simulink model "MC33pwm"  (R2019a)
settings: Solver=ode23tb  StartTime=0.0  StopTime=0.2  RelTol=1e-3
libraries: powerlib x35
(part 2 of 2)

== system MC33pwm/Subsystem1/status/time xl/time xl pos/xl b_u ==
  In ABC : Inport
  In x : Inport  Port=2
  Logical Operator : Logic  Operator=NOT  AllPortsSameDT=off  OutDataTypeStr=boolean
  MinMax : MinMax
  Sign : Signum
  Sum : Sum  Inputs=|+-
  out xl_s12 : Outport
  wires:
  Sign/1 -> Logical Operator/1
  MinMax/1 -> Sum/1
  Logical Operator/1 -> out xl_s12/1
  In ABC/1 -> MinMax/1
  In x/1 -> Sum/2
  Sum/1 -> Sign/1

== system MC33pwm/Subsystem1/status/time xl/time xl pos/xl c_u ==
  In ABC : Inport
  In x : Inport  Port=2
  Logical Operator : Logic  Operator=NOT  AllPortsSameDT=off  OutDataTypeStr=boolean
  MinMax : MinMax
  Sign : Signum
  Sum : Sum  Inputs=|+-
  out xl_s13 : Outport
  wires:
  Sign/1 -> Logical Operator/1
  MinMax/1 -> Sum/1
  Logical Operator/1 -> out xl_s13/1
  In ABC/1 -> MinMax/1
  In x/1 -> Sum/2
  Sum/1 -> Sign/1

== system MC33pwm/Subsystem1/status/time zb/time zb neg/zb a_u ==
  In ABC : Inport
  In x : Inport  Port=2
  Logical Operator : Logic  Operator=NOT  AllPortsSameDT=off  OutDataTypeStr=boolean
  MinMax : MinMax  Function=max
  Sign : Signum
  Sum : Sum  Inputs=|+-
  out zb_s11 : Outport
  wires:
  MinMax/1 -> Sum/1
  In ABC/1 -> MinMax/1
  In x/1 -> Sum/2
  Sum/1 -> Sign/1
  Sign/1 -> Logical Operator/1
  Logical Operator/1 -> out zb_s11/1

== system MC33pwm/Subsystem1/status/time zb/time zb neg/zb b_u ==
  In ABC : Inport
  In x : Inport  Port=2
  Logical Operator : Logic  Operator=NOT  AllPortsSameDT=off  OutDataTypeStr=boolean
  MinMax : MinMax  Function=max
  Sign : Signum
  Sum : Sum  Inputs=|+-
  out zb_s12 : Outport
  wires:
  MinMax/1 -> Sum/1
  In ABC/1 -> MinMax/1
  In x/1 -> Sum/2
  Sum/1 -> Sign/1
  Logical Operator/1 -> out zb_s12/1
  Sign/1 -> Logical Operator/1

== system MC33pwm/Subsystem1/status/time zb/time zb neg/zb c_u ==
  In ABC : Inport
  In x : Inport  Port=2
  Logical Operator : Logic  Operator=NOT  AllPortsSameDT=off  OutDataTypeStr=boolean
  MinMax : MinMax  Function=max
  Sign : Signum
  Sum : Sum  Inputs=|+-
  out zb_s13 : Outport
  wires:
  MinMax/1 -> Sum/1
  In ABC/1 -> MinMax/1
  In x/1 -> Sum/2
  Sum/1 -> Sign/1
  Logical Operator/1 -> out zb_s13/1
  Sign/1 -> Logical Operator/1

== system MC33pwm/Subsystem1/status/time zb/time zb pos/zb a_u ==
  In ABC : Inport
  In x : Inport  Port=2
  Logical Operator : Logic  Operator=NOT  AllPortsSameDT=off  OutDataTypeStr=boolean
  MinMax : MinMax  Function=max
  Scope : Scope
  Sign : Signum
  Sum : Sum  Inputs=|+-
  out zb_s11 : Outport
  wires:
  Sign/1 -> Logical Operator/1
  MinMax/1 -> Sum/1
  Logical Operator/1 -> out zb_s11/1
  In ABC/1 -> MinMax/1
  In x/1 -> Sum/2
  Sum/1 -> Scope/1, Sign/1

== system MC33pwm/Subsystem1/status/time zb/time zb pos/zb b_u ==
  In ABC : Inport
  In x : Inport  Port=2
  Logical Operator : Logic  Operator=NOT  AllPortsSameDT=off  OutDataTypeStr=boolean
  MinMax : MinMax  Function=max
  Sign : Signum
  Sum : Sum  Inputs=|+-
  out zb_s12 : Outport
  wires:
  Sign/1 -> Logical Operator/1
  MinMax/1 -> Sum/1
  Logical Operator/1 -> out zb_s12/1
  In ABC/1 -> MinMax/1
  In x/1 -> Sum/2
  Sum/1 -> Sign/1

== system MC33pwm/Subsystem1/status/time zb/time zb pos/zb c_u ==
  In ABC : Inport
  In x : Inport  Port=2
  Logical Operator : Logic  Operator=NOT  AllPortsSameDT=off  OutDataTypeStr=boolean
  MinMax : MinMax  Function=max
  Sign : Signum
  Sum : Sum  Inputs=|+-
  out zb_s13 : Outport
  wires:
  Sign/1 -> Logical Operator/1
  MinMax/1 -> Sum/1
  Logical Operator/1 -> out zb_s13/1
  In ABC/1 -> MinMax/1
  In x/1 -> Sum/2
  Sum/1 -> Sign/1

== system MC33pwm/Subsystem2/status/time xl/time xl neg/xl a_u ==
  In ABC : Inport
  In x : Inport  Port=2
  Logical Operator : Logic  Operator=NOT  AllPortsSameDT=off  OutDataTypeStr=boolean
  MinMax : MinMax
  Sign : Signum
  Sum : Sum  Inputs=|+-
  out xl_s11 : Outport
  wires:
  MinMax/1 -> Sum/1
  In ABC/1 -> MinMax/1
  In x/1 -> Sum/2
  Sum/1 -> Sign/1
  Sign/1 -> Logical Operator/1
  Logical Operator/1 -> out xl_s11/1

== system MC33pwm/Subsystem2/status/time xl/time xl neg/xl b_u ==
  In ABC : Inport
  In x : Inport  Port=2
  Logical Operator : Logic  Operator=NOT  AllPortsSameDT=off  OutDataTypeStr=boolean
  MinMax : MinMax
  Sign : Signum
  Sum : Sum  Inputs=|+-
  out xl_s12 : Outport
  wires:
  MinMax/1 -> Sum/1
  In ABC/1 -> MinMax/1
  In x/1 -> Sum/2
  Sum/1 -> Sign/1
  Logical Operator/1 -> out xl_s12/1
  Sign/1 -> Logical Operator/1

== system MC33pwm/Subsystem2/status/time xl/time xl neg/xl c_u ==
  In ABC : Inport
  In x : Inport  Port=2
  Logical Operator : Logic  Operator=NOT  AllPortsSameDT=off  OutDataTypeStr=boolean
  MinMax : MinMax
  Sign : Signum
  Sum : Sum  Inputs=|+-
  out xl_s13 : Outport
  wires:
  MinMax/1 -> Sum/1
  In ABC/1 -> MinMax/1
  In x/1 -> Sum/2
  Sum/1 -> Sign/1
  Logical Operator/1 -> out xl_s13/1
  Sign/1 -> Logical Operator/1

== system MC33pwm/Subsystem2/status/time xl/time xl pos/xl a_u ==
  In ABC : Inport
  In x : Inport  Port=2
  Logical Operator : Logic  Operator=NOT  AllPortsSameDT=off  OutDataTypeStr=boolean
  MinMax : MinMax
  Scope : Scope
  Sign : Signum
  Sum : Sum  Inputs=|+-
  out xl_s11 : Outport
  wires:
  Sign/1 -> Logical Operator/1
  MinMax/1 -> Sum/1
  Logical Operator/1 -> out xl_s11/1
  In ABC/1 -> MinMax/1
  In x/1 -> Sum/2
  Sum/1 -> Scope/1, Sign/1

== system MC33pwm/Subsystem2/status/time xl/time xl pos/xl b_u ==
  In ABC : Inport
  In x : Inport  Port=2
  Logical Operator : Logic  Operator=NOT  AllPortsSameDT=off  OutDataTypeStr=boolean
  MinMax : MinMax
  Sign : Signum
  Sum : Sum  Inputs=|+-
  out xl_s12 : Outport
  wires:
  Sign/1 -> Logical Operator/1
  MinMax/1 -> Sum/1
  Logical Operator/1 -> out xl_s12/1
  In ABC/1 -> MinMax/1
  In x/1 -> Sum/2
  Sum/1 -> Sign/1

== system MC33pwm/Subsystem2/status/time xl/time xl pos/xl c_u ==
  In ABC : Inport
  In x : Inport  Port=2
  Logical Operator : Logic  Operator=NOT  AllPortsSameDT=off  OutDataTypeStr=boolean
  MinMax : MinMax
  Sign : Signum
  Sum : Sum  Inputs=|+-
  out xl_s13 : Outport
  wires:
  Sign/1 -> Logical Operator/1
  MinMax/1 -> Sum/1
  Logical Operator/1 -> out xl_s13/1
  In ABC/1 -> MinMax/1
  In x/1 -> Sum/2
  Sum/1 -> Sign/1

== system MC33pwm/Subsystem2/status/time zb/time zb neg/zb a_u ==
  In ABC : Inport
  In x : Inport  Port=2
  Logical Operator : Logic  Operator=NOT  AllPortsSameDT=off  OutDataTypeStr=boolean
  MinMax : MinMax  Function=max
  Sign : Signum
  Sum : Sum  Inputs=|+-
  out zb_s11 : Outport
  wires:
  MinMax/1 -> Sum/1
  In ABC/1 -> MinMax/1
  In x/1 -> Sum/2
  Sum/1 -> Sign/1
  Sign/1 -> Logical Operator/1
  Logical Operator/1 -> out zb_s11/1

== system MC33pwm/Subsystem2/status/time zb/time zb neg/zb b_u ==
  In ABC : Inport
  In x : Inport  Port=2
  Logical Operator : Logic  Operator=NOT  AllPortsSameDT=off  OutDataTypeStr=boolean
  MinMax : MinMax  Function=max
  Sign : Signum
  Sum : Sum  Inputs=|+-
  out zb_s12 : Outport
  wires:
  MinMax/1 -> Sum/1
  In ABC/1 -> MinMax/1
  In x/1 -> Sum/2
  Sum/1 -> Sign/1
  Logical Operator/1 -> out zb_s12/1
  Sign/1 -> Logical Operator/1

== system MC33pwm/Subsystem2/status/time zb/time zb neg/zb c_u ==
  In ABC : Inport
  In x : Inport  Port=2
  Logical Operator : Logic  Operator=NOT  AllPortsSameDT=off  OutDataTypeStr=boolean
  MinMax : MinMax  Function=max
  Sign : Signum
  Sum : Sum  Inputs=|+-
  out zb_s13 : Outport
  wires:
  MinMax/1 -> Sum/1
  In ABC/1 -> MinMax/1
  In x/1 -> Sum/2
  Sum/1 -> Sign/1
  Logical Operator/1 -> out zb_s13/1
  Sign/1 -> Logical Operator/1

== system MC33pwm/Subsystem2/status/time zb/time zb pos/zb a_u ==
  In ABC : Inport
  In x : Inport  Port=2
  Logical Operator : Logic  Operator=NOT  AllPortsSameDT=off  OutDataTypeStr=boolean
  MinMax : MinMax  Function=max
  Scope : Scope
  Sign : Signum
  Sum : Sum  Inputs=|+-
  out zb_s11 : Outport
  wires:
  Sign/1 -> Logical Operator/1
  MinMax/1 -> Sum/1
  Logical Operator/1 -> out zb_s11/1
  In ABC/1 -> MinMax/1
  In x/1 -> Sum/2
  Sum/1 -> Scope/1, Sign/1

== system MC33pwm/Subsystem2/status/time zb/time zb pos/zb b_u ==
  In ABC : Inport
  In x : Inport  Port=2
  Logical Operator : Logic  Operator=NOT  AllPortsSameDT=off  OutDataTypeStr=boolean
  MinMax : MinMax  Function=max
  Sign : Signum
  Sum : Sum  Inputs=|+-
  out zb_s12 : Outport
  wires:
  Sign/1 -> Logical Operator/1
  MinMax/1 -> Sum/1
  Logical Operator/1 -> out zb_s12/1
  In ABC/1 -> MinMax/1
  In x/1 -> Sum/2
  Sum/1 -> Sign/1

== system MC33pwm/Subsystem2/status/time zb/time zb pos/zb c_u ==
  In ABC : Inport
  In x : Inport  Port=2
  Logical Operator : Logic  Operator=NOT  AllPortsSameDT=off  OutDataTypeStr=boolean
  MinMax : MinMax  Function=max
  Sign : Signum
  Sum : Sum  Inputs=|+-
  out zb_s13 : Outport
  wires:
  Sign/1 -> Logical Operator/1
  MinMax/1 -> Sum/1
  Logical Operator/1 -> out zb_s13/1
  In ABC/1 -> MinMax/1
  In x/1 -> Sum/2
  Sum/1 -> Sign/1

== system MC33pwm/Subsystem3/status/time xl/time xl neg/xl a_u ==
  In ABC : Inport
  In x : Inport  Port=2
  Logical Operator : Logic  Operator=NOT  AllPortsSameDT=off  OutDataTypeStr=boolean
  MinMax : MinMax
  Sign : Signum
  Sum : Sum  Inputs=|+-
  out xl_s11 : Outport
  wires:
  MinMax/1 -> Sum/1
  In ABC/1 -> MinMax/1
  In x/1 -> Sum/2
  Sum/1 -> Sign/1
  Sign/1 -> Logical Operator/1
  Logical Operator/1 -> out xl_s11/1

== system MC33pwm/Subsystem3/status/time xl/time xl neg/xl b_u ==
  In ABC : Inport
  In x : Inport  Port=2
  Logical Operator : Logic  Operator=NOT  AllPortsSameDT=off  OutDataTypeStr=boolean
  MinMax : MinMax
  Sign : Signum
  Sum : Sum  Inputs=|+-
  out xl_s12 : Outport
  wires:
  MinMax/1 -> Sum/1
  In ABC/1 -> MinMax/1
  In x/1 -> Sum/2
  Sum/1 -> Sign/1
  Logical Operator/1 -> out xl_s12/1
  Sign/1 -> Logical Operator/1

== system MC33pwm/Subsystem3/status/time xl/time xl neg/xl c_u ==
  In ABC : Inport
  In x : Inport  Port=2
  Logical Operator : Logic  Operator=NOT  AllPortsSameDT=off  OutDataTypeStr=boolean
  MinMax : MinMax
  Sign : Signum
  Sum : Sum  Inputs=|+-
  out xl_s13 : Outport
  wires:
  MinMax/1 -> Sum/1
  In ABC/1 -> MinMax/1
  In x/1 -> Sum/2
  Sum/1 -> Sign/1
  Logical Operator/1 -> out xl_s13/1
  Sign/1 -> Logical Operator/1

== system MC33pwm/Subsystem3/status/time xl/time xl pos/xl a_u ==
  In ABC : Inport
  In x : Inport  Port=2
  Logical Operator : Logic  Operator=NOT  AllPortsSameDT=off  OutDataTypeStr=boolean
  MinMax : MinMax
  Scope : Scope
  Sign : Signum
  Sum : Sum  Inputs=|+-
  out xl_s11 : Outport
  wires:
  Sign/1 -> Logical Operator/1
  MinMax/1 -> Sum/1
  Logical Operator/1 -> out xl_s11/1
  In ABC/1 -> MinMax/1
  In x/1 -> Sum/2
  Sum/1 -> Scope/1, Sign/1

== system MC33pwm/Subsystem3/status/time xl/time xl pos/xl b_u ==
  In ABC : Inport
  In x : Inport  Port=2
  Logical Operator : Logic  Operator=NOT  AllPortsSameDT=off  OutDataTypeStr=boolean
  MinMax : MinMax
  Sign : Signum
  Sum : Sum  Inputs=|+-
  out xl_s12 : Outport
  wires:
  Sign/1 -> Logical Operator/1
  MinMax/1 -> Sum/1
  Logical Operator/1 -> out xl_s12/1
  In ABC/1 -> MinMax/1
  In x/1 -> Sum/2
  Sum/1 -> Sign/1

== system MC33pwm/Subsystem3/status/time xl/time xl pos/xl c_u ==
  In ABC : Inport
  In x : Inport  Port=2
  Logical Operator : Logic  Operator=NOT  AllPortsSameDT=off  OutDataTypeStr=boolean
  MinMax : MinMax
  Sign : Signum
  Sum : Sum  Inputs=|+-
  out xl_s13 : Outport
  wires:
  Sign/1 -> Logical Operator/1
  MinMax/1 -> Sum/1
  Logical Operator/1 -> out xl_s13/1
  In ABC/1 -> MinMax/1
  In x/1 -> Sum/2
  Sum/1 -> Sign/1

== system MC33pwm/Subsystem3/status/time zb/time zb neg/zb a_u ==
  In ABC : Inport
  In x : Inport  Port=2
  Logical Operator : Logic  Operator=NOT  AllPortsSameDT=off  OutDataTypeStr=boolean
  MinMax : MinMax  Function=max
  Sign : Signum
  Sum : Sum  Inputs=|+-
  out zb_s11 : Outport
  wires:
  MinMax/1 -> Sum/1
  In ABC/1 -> MinMax/1
  In x/1 -> Sum/2
  Sum/1 -> Sign/1
  Sign/1 -> Logical Operator/1
  Logical Operator/1 -> out zb_s11/1

== system MC33pwm/Subsystem3/status/time zb/time zb neg/zb b_u ==
  In ABC : Inport
  In x : Inport  Port=2
  Logical Operator : Logic  Operator=NOT  AllPortsSameDT=off  OutDataTypeStr=boolean
  MinMax : MinMax  Function=max
  Sign : Signum
  Sum : Sum  Inputs=|+-
  out zb_s12 : Outport
  wires:
  MinMax/1 -> Sum/1
  In ABC/1 -> MinMax/1
  In x/1 -> Sum/2
  Sum/1 -> Sign/1
  Logical Operator/1 -> out zb_s12/1
  Sign/1 -> Logical Operator/1

== system MC33pwm/Subsystem3/status/time zb/time zb neg/zb c_u ==
  In ABC : Inport
  In x : Inport  Port=2
  Logical Operator : Logic  Operator=NOT  AllPortsSameDT=off  OutDataTypeStr=boolean
  MinMax : MinMax  Function=max
  Sign : Signum
  Sum : Sum  Inputs=|+-
  out zb_s13 : Outport
  wires:
  MinMax/1 -> Sum/1
  In ABC/1 -> MinMax/1
  In x/1 -> Sum/2
  Sum/1 -> Sign/1
  Logical Operator/1 -> out zb_s13/1
  Sign/1 -> Logical Operator/1

== system MC33pwm/Subsystem3/status/time zb/time zb pos/zb a_u ==
  In ABC : Inport
  In x : Inport  Port=2
  Logical Operator : Logic  Operator=NOT  AllPortsSameDT=off  OutDataTypeStr=boolean
  MinMax : MinMax  Function=max
  Scope : Scope
  Sign : Signum
  Sum : Sum  Inputs=|+-
  out zb_s11 : Outport
  wires:
  Sign/1 -> Logical Operator/1
  MinMax/1 -> Sum/1
  Logical Operator/1 -> out zb_s11/1
  In ABC/1 -> MinMax/1
  In x/1 -> Sum/2
  Sum/1 -> Scope/1, Sign/1

== system MC33pwm/Subsystem3/status/time zb/time zb pos/zb b_u ==
  In ABC : Inport
  In x : Inport  Port=2
  Logical Operator : Logic  Operator=NOT  AllPortsSameDT=off  OutDataTypeStr=boolean
  MinMax : MinMax  Function=max
  Sign : Signum
  Sum : Sum  Inputs=|+-
  out zb_s12 : Outport
  wires:
  Sign/1 -> Logical Operator/1
  MinMax/1 -> Sum/1
  Logical Operator/1 -> out zb_s12/1
  In ABC/1 -> MinMax/1
  In x/1 -> Sum/2
  Sum/1 -> Sign/1

== system MC33pwm/Subsystem3/status/time zb/time zb pos/zb c_u ==
  In ABC : Inport
  In x : Inport  Port=2
  Logical Operator : Logic  Operator=NOT  AllPortsSameDT=off  OutDataTypeStr=boolean
  MinMax : MinMax  Function=max
  Sign : Signum
  Sum : Sum  Inputs=|+-
  out zb_s13 : Outport
  wires:
  Sign/1 -> Logical Operator/1
  MinMax/1 -> Sum/1
  Logical Operator/1 -> out zb_s13/1
  In ABC/1 -> MinMax/1
  In x/1 -> Sum/2
  Sum/1 -> Sign/1
